simulink model "CT_2"  (Simulink 8.1)
settings: Solver=ode45  StartTime=0.0  StopTime=10e-6  RelTol=1e-3
libraries: commseqgen2 x1, commutil2 x1
settings Model: Creator=Мама Люда  LastModifiedBy=User
settings OptimizationCC: InitFltsAndDblsToZero=on
settings DebuggingCC: SaveWithParameterizedLinksMsg=none  StrictBusMsg=Warning
settings GRTTargetCC: TargetFcnLib=ansi_tfl_tmw.mat

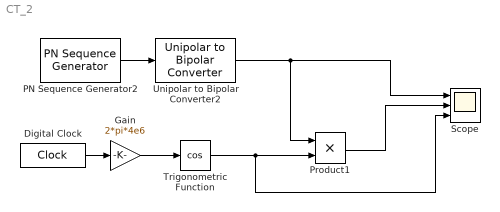
== system CT_2 ==
  Digital Clock : DigitalClock  SampleTime=1e-8
  Gain : Gain  Gain=2*pi*4e6
  PN Sequence Generator2 : commseqgen2/PN Sequence Generator  poly=[1 0 0 0 0 1 0 0 0 1]  ini_sta=[1 1 1 1 1 1 1 0 1]  outBitMaskSource=Dialog parameter  shift=0  outVarSiz=off  maxOutSizeMode=Dialog parameter  maxOutSize=[10 1]  Ts=1.955e-6  frameBased=off  sampPerFrame=1  reset=off  bitPackedOutputs=off  outDataType=boolean  numPackedBits=8  bitPackDataSigned=off  bitPackedOutDType=double
  Product1 : Product  RndMeth=Zero
  Scope : Scope  NumInputPorts=3
      settings: TimeRange=4e-05  YMin=-2~-2~-5  YMax=2~2~5  SampleInput=on  SampleTime=1e-8
  Trigonometric Function : Trigonometry  Operator=cos
  Unipolar to Bipolar Converter2 : commutil2/Unipolar to Bipolar Converter  M=2  polarity=Positive  dataType=double
  wires:
  Unipolar to Bipolar Converter2/1 -> Scope/1, Product1/1
  PN Sequence Generator2/1 -> Unipolar to Bipolar Converter2/1
  Digital Clock/1 -> Gain/1
  Gain/1 -> Trigonometric Function/1
  Product1/1 -> Scope/2
  Trigonometric Function/1 -> Scope/3, Product1/2
